simulink model "martalg2"  (R2013a)
settings: Solver=ode45  StartTime=0.0  StopTime=10.0  RelTol=1e-3
settings Model: ExtModeAutoUpdateStatusClock=off  Creator=pmosterm  LastModifiedBy=sshringa
settings DataIOCC: SaveFormat=StructureWithTime  SignalLoggingSaveFormat=ModelDataLogs  SignalLoggingName=logsOut
settings OptimizationCC: InlineParams=on  InlineInvariantSignals=on  InitFltsAndDblsToZero=on
settings DebuggingCC: SaveWithParameterizedLinksMsg=none  SignalResolutionControl=TryResolveAllWithWarning  SolverPrmCheckMsg=none  MultiTaskDSMMsg=warning  MultiTaskCondExecSysMsg=none  FcnCallInpInsideContextMsg=UseLocalSettings
settings ModelReferenceCC: ModelReferenceMinAlgLoopOccurrences=on
settings RTWCC: ProcessScript=grt_make_rtw_hook  IncludeERTFirstTime=on

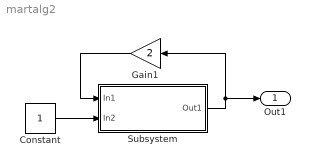
== system martalg2 ==
  Constant : Constant  SampleTime=1
  Gain1 : Gain  Gain=2
  Subsystem : Subsystem  TreatAsAtomicUnit=on
      settings: MinAlgLoopOccurrences=on
  Out1 : Outport
  wires:
  Subsystem/1(Out1) -> Gain1/1, Out1/1
  Constant/1 -> Subsystem/2(In2)
  Gain1/1 -> Subsystem/1(In1)

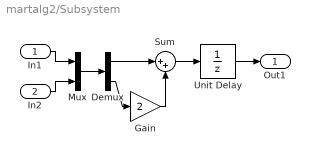
== system martalg2/Subsystem ==
  In1 : Inport
  In2 : Inport  Port=2
  Demux : Demux  Outputs=2
  Gain : Gain  Gain=2
  Mux : Mux  Inputs=2
  Sum : Sum  Inputs=|++
  Unit Delay : UnitDelay
  Out1 : Outport
  wires:
  Sum/1 -> Unit Delay/1
  Demux/1 -> Sum/1
  Gain/1 -> Sum/2
  Demux/2 -> Gain/1
  Mux/1 -> Demux/1
  In1/1 -> Mux/1
  Unit Delay/1 -> Out1/1
  In2/1 -> Mux/2
